simulink model "satellite3"  (R2025b)
settings: Solver=FixedStepAuto  StartTime=0.0  StopTime=100  FixedStep=dt  MinStep=0.0001  RelTol=1e-3
values from neighbouring files (symbols this model uses):
  A_mw = [ ... (first row only)    [init_params.m]
  A_w = [ ... (first row only)    [init_params.m]
  alpha1 = 0.1    [init_params.m]
  alpha2 = 0.1    [init_params.m]
  angle0 = eAR'    [init_params.m]
  area_d = 4    [init_params.m]
  area_m2 = 0.0127    [init_params.m]
  area_s = 2    [init_params.m]
  ARW_deg_per_sqrt_h = 0.01    [init_params.m]
  B_mw = [ ... (first row only)    [init_params.m]
  bat_bias_on = 0    [init_params.m]
  bat_bias_time = 0    [init_params.m]
  bat_bias_value = 0    [init_params.m]
  bat_cap_on = 0    [init_params.m]
  bat_cap_time = 0    [init_params.m]
  bat_cap_value = 1    [init_params.m]
  beta = 0.3    [init_params.m]
  beta1 = 0.01    [init_params.m]
  beta2 = 0.01    [init_params.m]
  bias0_deg_h = 0.01    [init_params.m]
  C_mw = [ ... (first row only)    [init_params.m]
  Cd = 2.2    [init_params.m]
  Cm = 0.01    [init_params.m]
  cmd_comm = 1    [init_params.m]
  comm_allow = 1    [init_params.m]
  cos_g_max = cos(gamma_max)    [init_params.m]
  Cr = 1.2    [init_params.m]
  cT_deg_on = 0    [init_params.m]
  cT_deg_time = 0    [init_params.m]
  cT_deg_value = 1    [init_params.m]
  cT_delay_on = 0    [init_params.m]
  cT_delay_time = 0    [init_params.m]
  cT_delay_value = 0    [init_params.m]
  cT_drop_on = 0    [init_params.m]
  cT_drop_time = 0    [init_params.m]
  cT_drop_value = 0    [init_params.m]
  cT_lock_on = 0    [init_params.m]
  cT_lock_time = 0    [init_params.m]
  d_c = 2e-5    (= 2e-05)    [init_params.m]
  d_f = 2e-5    (= 2e-05)    [init_params.m]
  D_max = 1    [init_params.m]
  D_thr = 0.4    [init_params.m]
  Delta_D = 0.001    [init_params.m]
  dP_th = 0.05    [init_params.m]
  dss_bias_on = 0    [init_params.m]
  dss_bias_time = 0    [init_params.m]
  dss_bias_value = [0;0;0]    [init_params.m]
  dss_delay_on = 0    [init_params.m]
  dss_delay_time = 0    [init_params.m]
  dss_delay_value = 0    [init_params.m]
  dss_drift_max = 0.1    [init_params.m]
  dss_drift_value = [0;0;0]    [init_params.m]
  dss_drop_on = 0    [init_params.m]
  dss_drop_time = 0    [init_params.m]
  dss_drop_value = [1;0;0]    [init_params.m]
  dss_lock_on = 0    [init_params.m]
  dss_lock_time = 0    [init_params.m]
  dt = 0.1    [init_params.m]
  earth_theta0 = 0    [init_params.m]
  epsilon = 0.01    [init_params.m]
  eT_deg_on = 0    [init_params.m]
  eT_deg_time = 0    [init_params.m]
  eT_deg_value = 1    [init_params.m]
  eT_delay_on = 0    [init_params.m]
  eT_delay_time = 0    [init_params.m]
  eT_delay_value = 0    [init_params.m]
  eT_drop_on = 0    [init_params.m]
  eT_drop_time = 0    [init_params.m]
  eT_drop_value = [0;0;0]    [init_params.m]
  eT_lock_on = 0    [init_params.m]
  eT_lock_time = 0    [init_params.m]
  eta = 0.7    [init_params.m]
  eta_buck = 0.9    [init_params.m]
  eta_et = 0.9    [init_params.m]
  eta_sspa = 0.35    [init_params.m]
  eta_twta = 0.35    [init_params.m]
  f = 2.2e9    (= 2200000000)    [init_params.m]
  f_n_hz = 400    [init_params.m]
  fov = 60*pi/180    (= 1.0471975512)    [init_params.m]
  g0 = 9.80665    [init_params.m]
  G0 = 1366.1    [init_params.m]
  G_sspa_dB = 20    [init_params.m]
  G_twta_dB = 20    [init_params.m]
  Gr_dB = 20    [init_params.m]
  Gt_dB = 3    [init_params.m]
  gyro_bias_on = 0    [init_params.m]
  gyro_bias_time = 0    [init_params.m]
  gyro_bias_value = [0;0;0]    [init_params.m]
  gyro_delay_on = 0    [init_params.m]
  gyro_delay_time = 0    [init_params.m]
  gyro_delay_value = 0    [init_params.m]
  gyro_drift_max = 0.1    [init_params.m]
  gyro_drift_value = [0;0;0]    [init_params.m]
  gyro_drop_on = 0    [init_params.m]
  gyro_drop_time = 0    [init_params.m]
  gyro_drop_value = [0;0;0]    [init_params.m]
  gyro_lock_on = 0    [init_params.m]
  gyro_lock_time = 0    [init_params.m]
  H = 50e3    (= 50000)    [init_params.m]
  h_max = Iw * rpm_max * sqrt(6)    [init_params.m]
  h_ref = 400e3    (= 400000)    [init_params.m]
  I_e = 11    [init_params.m]
  I_gate = 0.5    [init_params.m]
  I_triggle = 8    [init_params.m]
  i_w_max = 2    [init_params.m]
  i_w_min = -2    [init_params.m]
  initial_phase = 0    [init_params.m]
  Isp = 220    [init_params.m]
  Isp_et = 1500    [init_params.m]
  Iw = 0.02    [init_params.m]
  J2 = 1.08262668e-3    (= 0.00108262668)    [init_params.m]
  Jx = 10    [init_params.m]
  Jy = 12    [init_params.m]
  Jz = 8    [init_params.m]
  k_a = 4e-4    (= 0.0004)    [init_params.m]
  k_bias1_deg_h_per_C = 1    [init_params.m]
  k_bias2_deg_h_per_C = 0.0    (= 0)    [init_params.m]
  k_h = -0.05    [init_params.m]
  k_sf1_ppm = 1.0    (= 1)    [init_params.m]
  k_sf2_ppm = 0.0    (= 0)    [init_params.m]
  ... (+207 more)
libraries: matrix_library x25, simulink x14, nesl_utility x4, simulink_extras x3, fl_lib x3, ee_lib x1
(part 3 of 5)

== system satellite3/姿态确定与控制系统/三轴姿态动力学子系统/rlg_q/控模与扫模逻辑 ==
  光强 : Inport
  Add : Sum  Inputs=+-
  Add1 : Sum
  Gain : Gain  Gain=kP
  Gain1 : Gain  Gain=kI
  Integrator : Integrator
  Switch : Switch  Criteria=u2 > Threshold  SaturateOnIntegerOverflow=off  InputSameDT=off
  zero : Constant  Value=0  OutDataTypeStr=boolean
  光强阈值 : Constant  Value=I_triggle
  扫模信号发生器 : simulink/Sources/Repeating Sequence  rep_seq_t=[0 0.5 1]  rep_seq_y=[0 V_pzt_max V_pzt_min]
  期望光强 : Constant  Value=I_e
  状态切换 : simulink_extras/Flip Flops/S-R Flip-Flop  initial_condition=0
  触发信号 : RelationalOperator  OutDataTypeStr=boolean  RndMeth=Simplest  InputSameDT=off
  触发信号1 : RelationalOperator  Operator=<  OutDataTypeStr=boolean  RndMeth=Simplest  InputSameDT=off
  跌落阈值 : Constant  Value=I_gate
  扫模电压 : Outport
  wires:
  跌落阈值/1 -> 触发信号1/2
  光强/1 -> 触发信号/1, Add/2, 触发信号1/1
  触发信号1/1 -> 状态切换/2
  Integrator/1 -> Add1/1
  Gain1/1 -> Integrator/1
  Gain/1 -> Add1/2
  Add/1 -> Gain/1, Gain1/1
  Switch/1 -> 扫模电压/1
  触发信号/1 -> 状态切换/1
  扫模信号发生器/1 -> Switch/3
  状态切换/1 -> Switch/2
  Add1/1 -> Switch/1
  期望光强/1 -> Add/1
  光强阈值/1 -> 触发信号/2

== system satellite3/姿态确定与控制系统/三轴姿态动力学子系统/rlg_q/机械抖动 ==
  Add : Sum
  Add1 : Sum  Inputs=-+-
  Clock : Clock
  Product{,1..3,5} (5 alike) : Product
  Product6 : Product  Inputs=3
  Scope : Scope
      settings: DataLoggingVariableName=ScopeData4
  Scope1 : Scope
      settings: DataLoggingVariableName=ScopeData5
  Sin : Trigonometry
  Square : Math  Operator=square
  deg2rad : Gain  Gain=pi/180
  dither_d : ToWorkspace  VariableName=dither_d  SampleTime=-1
  dither_w : ToWorkspace  VariableName=dither_w  SampleTime=-1
  r2rad : Gain  Gain=2*pi
  倍数 : Constant  Value=2.0
  初相位 : Constant  Value=initial_phase
  抖动固有频率-Hz : Constant  Value=f_n_hz
  抖动角度迭代 : Integrator
  抖动角速度迭代 : Integrator
  抖动角速度（峰值）-deg/s : Constant  Value=v_peak_deg_s
  阻尼比 : Constant  Value=zeta
  抖动角速度 : Outport
  wires:
  抖动角速度迭代/1 -> 抖动角度迭代/1, 抖动角速度/1, Product6/3, dither_w/1, Scope/1
  Product5/1 -> Add1/1
  抖动角度迭代/1 -> Product5/1, Scope1/1, dither_d/1
  Square/1 -> Product5/2
  Product6/1 -> Add1/3
  Add1/1 -> 抖动角速度迭代/1
  Product/1 -> Product3/2, Product6/2
  抖动角速度（峰值）-deg/s/1 -> deg2rad/1
  deg2rad/1 -> Product3/1  "抖动角度幅值-rad"
  Product2/1 -> Add1/2  "驱动力矩-N·m"
  Sin/1 -> Product2/2
  Product3/1 -> Product2/1  "驱动力矩幅值-N·m"
  Add/1 -> Sin/1
  初相位/1 -> Add/2
  Product1/1 -> Add/1
  Clock/1 -> Product1/1
  倍数/1 -> Product/1
  阻尼比/1 -> Product/2
  抖动固有频率-Hz/1 -> r2rad/1
  r2rad/1 -> Product1/2, Product6/1, Square/1  "抖动固有角频率-rad/s"

== system satellite3/姿态确定与控制系统/三轴姿态动力学子系统/rlg_q/热模型 ==
  环境温度-°C : Inport
  几何标度因数 : Inport  Port=2
  Add : Sum
  Add1 : Sum  Inputs=+++
  Add2 : Sum
  Product : Product
  Sum : Sum  Inputs=|-+
  deg2rad(s) : Gain  Gain=pi/(180*3600)
  平方 : Math  Operator=square
  标定/初始温度 : Constant  Value=25
  标度因数倍数（参考温度） : Constant
  比较 : Sum  Inputs=-+|
  温度标度因数系数（1阶） : Gain  Gain=k_sf1_ppm
  温度标度因数系数（2阶） : Gain  Gain=k_sf2_ppm
  温度迭代 : Integrator  InitialConditionSource=external  InitialCondition=25.0
  温度零偏系数（1阶） : Gain  Gain=k_bias1_deg_h_per_C
  温度零偏系数（2阶） : Gain  Gain=k_bias2_deg_h_per_C
  热时间常数 : Gain  Gain=1/tau_th_s
  百万分之一每摄氏度 : Gain  Gain=1e-6
  零偏（参考温度） : Constant  Value=bias0_deg_h
  陀螺温度-°C : Outport
  温度标度因数 : Outport  Port=2
  温度零偏 : Outport  Port=3
  wires:
  Add2/1 -> Product/2
  标度因数倍数（参考温度）/1 -> Add2/1
  百万分之一每摄氏度/1 -> Add2/2
  零偏（参考温度）/1 -> Add1/1
  温度零偏系数（1阶）/1 -> Add1/2
  温度零偏系数（2阶）/1 -> Add1/3
  Sum/1 -> 温度零偏系数（1阶）/1, 温度标度因数系数（1阶）/1, 平方/1
  Add1/1 -> deg2rad(s)/1
  几何标度因数/1 -> Product/1
  deg2rad(s)/1 -> 温度零偏/1
  平方/1 -> 温度零偏系数（2阶）/1, 温度标度因数系数（2阶）/1
  Product/1 -> 温度标度因数/1
  Add/1 -> 百万分之一每摄氏度/1
  标定/初始温度/1 -> 温度迭代/2, Sum/1
  温度标度因数系数（2阶）/1 -> Add/2
  温度标度因数系数（1阶）/1 -> Add/1
  比较/1 -> 热时间常数/1
  环境温度-°C/1 -> 比较/2
  温度迭代/1 -> 比较/1, Sum/2, 陀螺温度-°C/1
  热时间常数/1 -> 温度迭代/1

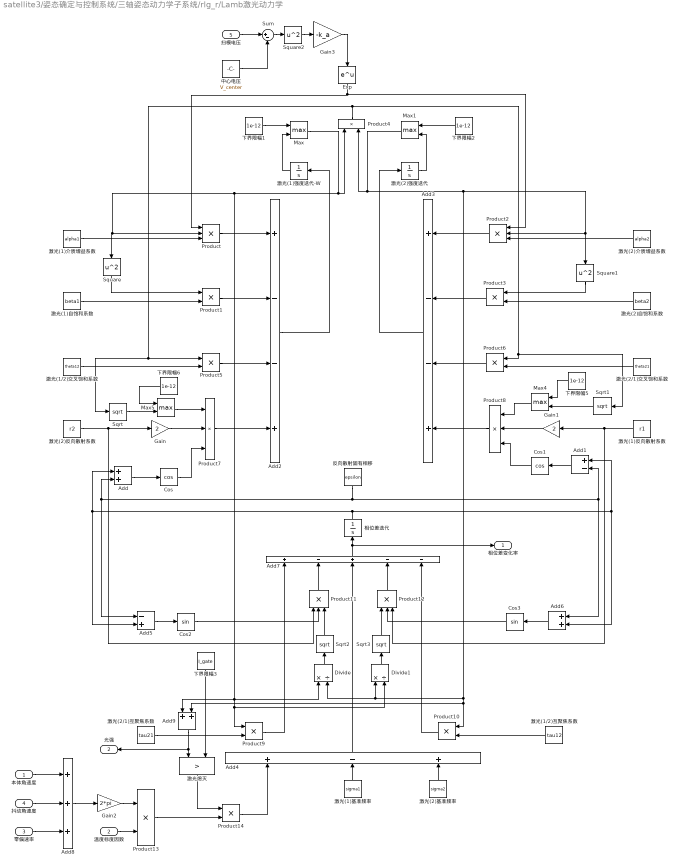
== system satellite3/姿态确定与控制系统/三轴姿态动力学子系统/rlg_r/Lamb激光动力学 ==
  本体角速度 : Inport
  温度标度因数 : Inport  Port=2
  零偏速率 : Inport  Port=3
  抖动角速度 : Inport  Port=4
  扫模电压 : Inport  Port=5
  Add : Sum
  Add1 : Sum  Inputs=+-
  Add2 : Sum  Inputs=+--+
  Add3 : Sum  Inputs=+--+
  Add4 : Sum  Inputs=+-+
  Add5 : Sum  Inputs=-+
  Add6 : Sum
  Add7 : Sum  Inputs=+-+--
  Add8 : Sum  Inputs=+++
  Add9 : Sum
  Cos : Trigonometry  Operator=cos
  Cos1 : Trigonometry  Operator=cos
  Cos2 : Trigonometry
  Cos3 : Trigonometry
  Divide : Product  Inputs=*/
  Divide1 : Product  Inputs=*/
  Exp : Math
  Gain : Gain  Gain=2
  Gain1 : Gain  Gain=2
  Gain2 : Gain  Gain=2*pi
  Gain3 : Gain  Gain=-k_a
  Max{,1,4..5} (4 alike) : MinMax  Function=max  Inputs=2
  Product{,2,7..8,11..12} (6 alike) : Product  Inputs=3
  Product{1,3..6,9..10,13..14} (9 alike) : Product
  Sqrt{,1..3} (4 alike) : Sqrt
  Square : Math  Operator=square
  Square1 : Math  Operator=square
  Square2 : Math  Operator=square
  Sum : Sum  Inputs=|+-
  下界限幅{1..2,5..6} (4 alike) : Constant  Value=1e-12
  下界限幅3 : Constant  Value=I_gate
  中心电压 : Constant  Value=V_center
  反向散射固有相移 : Constant  Value=epsilon
  激光(1)介质增益系数 : Constant  Value=alpha1
  激光(1)反向散射系数 : Constant  Value=r1
  激光(1)基准频率 : Constant  Value=sigma1
  激光(1)强度迭代-W : Integrator  InitialCondition=1
  激光(1)自饱和系数 : Constant  Value=beta1
  激光(1/2)互聚焦系数 : Constant  Value=tau12
  激光(1/2)交叉饱和系数 : Constant  Value=theta12
  激光(2)介质增益系数 : Constant  Value=alpha2
  激光(2)反向散射系数 : Constant  Value=r2
  激光(2)基准频率 : Constant  Value=sigma2
  激光(2)强度迭代 : Integrator  InitialCondition=1
  激光(2)自饱和系数 : Constant  Value=beta2
  激光(2/1)互聚焦系数 : Constant  Value=tau21
  激光(2/1)交叉饱和系数 : Constant  Value=theta21
  激光熄灭 : RelationalOperator  Operator=>  OutDataTypeStr=boolean  InputSameDT=off
  相位差迭代 : Integrator
  相位差变化率 : Outport
  光强 : Outport  Port=2
  wires:
  激光(1)介质增益系数/1 -> Product/3
  激光(1)自饱和系数/1 -> Product1/2
  Square/1 -> Product1/1
  激光(2)介质增益系数/1 -> Product2/3
  激光(2)自饱和系数/1 -> Product3/2
  Square1/1 -> Product3/1
  激光(1/2)交叉饱和系数/1 -> Product5/2
  激光(2/1)交叉饱和系数/1 -> Product6/2
  下界限幅1/1 -> Max/1
  Product4/1 -> Product6/1, Sqrt1/1, Product5/1, Sqrt/1
  激光(2)反向散射系数/1 -> Gain/1, Product11/1
  Gain/1 -> Product7/2
  Max5/1 -> Product7/1
  Cos/1 -> Product7/3
  Add/1 -> Cos/1
  反向散射固有相移/1 -> Add1/2, Add6/1, Add5/1, Add/2
  Cos1/1 -> Product8/3
  Max4/1 -> Product8/1
  Add1/1 -> Cos1/1
  Gain1/1 -> Product8/2
  激光(1)反向散射系数/1 -> Product12/3, Gain1/1
  下界限幅2/1 -> Max1/1
  Product/1 -> Add2/1
  Product1/1 -> Add2/2
  Product5/1 -> Add2/3
  Add2/1 -> 激光(1)强度迭代-W/1
  Product2/1 -> Add3/1
  Product3/1 -> Add3/2
  Product6/1 -> Add3/3
  Product8/1 -> Add3/4
  Add3/1 -> 激光(2)强度迭代/1
  激光(2/1)互聚焦系数/1 -> Product9/2
  激光(1/2)互聚焦系数/1 -> Product10/2
  Product7/1 -> Add2/4
  Add5/1 -> Cos2/1
  Max/1 -> Add9/1, Product9/1, Divide1/2, Divide/1, Product/2, Square/1, Product4/1
  Divide/1 -> Sqrt2/1
  Cos2/1 -> Product11/2
  相位差迭代/1 -> Add1/1, Add6/2, Add5/2, Add/1
  Add6/1 -> Cos3/1
  Divide1/1 -> Sqrt3/1
  Cos3/1 -> Product12/2
  激光(1)基准频率/1 -> Add4/2
  激光(2)基准频率/1 -> Add4/3
  Product14/1 -> Add4/1
  Product9/1 -> Add7/1
  Product10/1 -> Add7/5
  Product11/1 -> Add7/2
  Product12/1 -> Add7/4
  Add4/1 -> Add7/3
  Add7/1 -> 相位差变化率/1, 相位差迭代/1
  激光(1)强度迭代-W/1 -> Max/2
  激光(2)强度迭代/1 -> Max1/2
  下界限幅5/1 -> Max4/1
  Sqrt1/1 -> Max4/2
  下界限幅6/1 -> Max5/1
  Sqrt/1 -> Max5/2
  Sqrt2/1 -> Product11/3
  Sqrt3/1 -> Product12/1
  零偏速率/1 -> Add8/3
  温度标度因数/1 -> Product13/2
  本体角速度/1 -> Add8/1
  抖动角速度/1 -> Add8/2
  Add8/1 -> Gain2/1
  Gain2/1 -> Product13/1
  Max1/1 -> Product4/2, Square1/1, Product2/2, Divide/2, Divide1/1, Add9/2, Product10/1
  Add9/1 -> 光强/1, 激光熄灭/1
  Product13/1 -> Product14/2
  激光熄灭/1 -> Product14/1
  下界限幅3/1 -> 激光熄灭/2
  扫模电压/1 -> Sum/1
  中心电压/1 -> Sum/2
  Sum/1 -> Square2/1
  Gain3/1 -> Exp/1
  Exp/1 -> Product2/1, Product/1
  Square2/1 -> Gain3/1

== system satellite3/姿态确定与控制系统/三轴姿态动力学子系统/rlg_r/几何参数 ==
  Mux : Mux  Inputs=3
  激光波长-m : Constant  Value=wavelength_m
  环形腔周长-m : Constant  Value=perimeter_m
  环形腔面积-m2 : Constant  Value=area_m2
  计算集合标度因数-S0 : Fcn  Expr=4*u(1)/(u(2)*u(3))
  标度因数 : Outport
  wires:
  计算集合标度因数-S0/1 -> 标度因数/1
  Mux/1 -> 计算集合标度因数-S0/1
  环形腔面积-m2/1 -> Mux/1
  激光波长-m/1 -> Mux/2
  环形腔周长-m/1 -> Mux/3

== system satellite3/姿态确定与控制系统/三轴姿态动力学子系统/rlg_r/噪声模型 ==
  标度因数 : Inport
  相位差变化率 : Inport  Port=2
  Add : Sum
  Band-Limited White Noise : simulink/Sources/Band-Limited White Noise  Cov=[(ARW_deg_per_sqrt_h/60)^2 + white_rate_std_deg_s^2]  Ts=1  seed=[23341]
  Divide : Product  Inputs=/*
  Gain : Gain  Gain=pi/180
  r2Hz : Gain  Gain=1/(2*pi)
  测量角速度 : Outport
  wires:
  Add/1 -> 测量角速度/1
  r2Hz/1 -> Divide/2
  Gain/1 -> Add/1
  Band-Limited White Noise/1 -> Gain/1
  Divide/1 -> Add/2
  相位差变化率/1 -> r2Hz/1
  标度因数/1 -> Divide/1

== system satellite3/姿态确定与控制系统/三轴姿态动力学子系统/rlg_r/控模与扫模逻辑 ==
  光强 : Inport
  Add : Sum  Inputs=+-
  Add1 : Sum
  Gain : Gain  Gain=kP
  Gain1 : Gain  Gain=kI
  Integrator : Integrator
  Switch : Switch  Criteria=u2 > Threshold  SaturateOnIntegerOverflow=off  InputSameDT=off
  zero : Constant  Value=0  OutDataTypeStr=boolean
  光强阈值 : Constant  Value=I_triggle
  扫模信号发生器 : simulink/Sources/Repeating Sequence  rep_seq_t=[0 0.5 1]  rep_seq_y=[0 V_pzt_max V_pzt_min]
  期望光强 : Constant  Value=I_e
  状态切换 : simulink_extras/Flip Flops/S-R Flip-Flop  initial_condition=0
  触发信号 : RelationalOperator  OutDataTypeStr=boolean  RndMeth=Simplest  InputSameDT=off
  触发信号1 : RelationalOperator  Operator=<  OutDataTypeStr=boolean  RndMeth=Simplest  InputSameDT=off
  跌落阈值 : Constant  Value=I_gate
  扫模电压 : Outport
  wires:
  光强阈值/1 -> 触发信号/2
  期望光强/1 -> Add/1
  Add1/1 -> Switch/1
  状态切换/1 -> Switch/2
  扫模信号发生器/1 -> Switch/3
  触发信号/1 -> 状态切换/1
  Switch/1 -> 扫模电压/1
  Add/1 -> Gain1/1, Gain/1
  Gain/1 -> Add1/2
  Gain1/1 -> Integrator/1
  Integrator/1 -> Add1/1
  触发信号1/1 -> 状态切换/2
  光强/1 -> 触发信号1/1, Add/2, 触发信号/1
  跌落阈值/1 -> 触发信号1/2

== system satellite3/姿态确定与控制系统/三轴姿态动力学子系统/rlg_r/机械抖动 ==
  Add : Sum
  Add1 : Sum  Inputs=-+-
  Clock : Clock
  Product{,1..3,5} (5 alike) : Product
  Product6 : Product  Inputs=3
  Scope : Scope
      settings: DataLoggingVariableName=ScopeData4
  Scope1 : Scope
      settings: DataLoggingVariableName=ScopeData5
  Sin : Trigonometry
  Square : Math  Operator=square
  deg2rad : Gain  Gain=pi/180
  dither_d : ToWorkspace  VariableName=dither_d  SampleTime=-1
  dither_w : ToWorkspace  VariableName=dither_w  SampleTime=-1
  r2rad : Gain  Gain=2*pi
  倍数 : Constant  Value=2.0
  初相位 : Constant  Value=initial_phase
  抖动固有频率-Hz : Constant  Value=f_n_hz
  抖动角度迭代 : Integrator
  抖动角速度迭代 : Integrator
  抖动角速度（峰值）-deg/s : Constant  Value=v_peak_deg_s
  阻尼比 : Constant  Value=zeta
  抖动角速度 : Outport
  wires:
  r2rad/1 -> Square/1, Product6/1, Product1/2  "抖动固有角频率-rad/s"
  抖动固有频率-Hz/1 -> r2rad/1
  阻尼比/1 -> Product/2
  倍数/1 -> Product/1
  Clock/1 -> Product1/1
  Product1/1 -> Add/1
  初相位/1 -> Add/2
  Add/1 -> Sin/1
  Product3/1 -> Product2/1  "驱动力矩幅值-N·m"
  Sin/1 -> Product2/2
  Product2/1 -> Add1/2  "驱动力矩-N·m"
  deg2rad/1 -> Product3/1  "抖动角度幅值-rad"
  抖动角速度（峰值）-deg/s/1 -> deg2rad/1
  Product/1 -> Product6/2, Product3/2
  Add1/1 -> 抖动角速度迭代/1
  Product6/1 -> Add1/3
  Square/1 -> Product5/2
  抖动角度迭代/1 -> dither_d/1, Scope1/1, Product5/1
  Product5/1 -> Add1/1
  抖动角速度迭代/1 -> Scope/1, dither_w/1, Product6/3, 抖动角速度/1, 抖动角度迭代/1

== system satellite3/姿态确定与控制系统/三轴姿态动力学子系统/rlg_r/热模型 ==
  环境温度-°C : Inport
  几何标度因数 : Inport  Port=2
  Add : Sum
  Add1 : Sum  Inputs=+++
  Add2 : Sum
  Product : Product
  Sum : Sum  Inputs=|-+
  deg2rad(s) : Gain  Gain=pi/(180*3600)
  平方 : Math  Operator=square
  标定/初始温度 : Constant  Value=25
  标度因数倍数（参考温度） : Constant
  比较 : Sum  Inputs=-+|
  温度标度因数系数（1阶） : Gain  Gain=k_sf1_ppm
  温度标度因数系数（2阶） : Gain  Gain=k_sf2_ppm
  温度迭代 : Integrator  InitialConditionSource=external  InitialCondition=25.0
  温度零偏系数（1阶） : Gain  Gain=k_bias1_deg_h_per_C
  温度零偏系数（2阶） : Gain  Gain=k_bias2_deg_h_per_C
  热时间常数 : Gain  Gain=1/tau_th_s
  百万分之一每摄氏度 : Gain  Gain=1e-6
  零偏（参考温度） : Constant  Value=bias0_deg_h
  陀螺温度-°C : Outport
  温度标度因数 : Outport  Port=2
  温度零偏 : Outport  Port=3
  wires:
  热时间常数/1 -> 温度迭代/1
  温度迭代/1 -> 陀螺温度-°C/1, Sum/2, 比较/1
  环境温度-°C/1 -> 比较/2
  比较/1 -> 热时间常数/1
  温度标度因数系数（1阶）/1 -> Add/1
  温度标度因数系数（2阶）/1 -> Add/2
  标定/初始温度/1 -> Sum/1, 温度迭代/2
  Add/1 -> 百万分之一每摄氏度/1
  Product/1 -> 温度标度因数/1
  平方/1 -> 温度标度因数系数（2阶）/1, 温度零偏系数（2阶）/1
  deg2rad(s)/1 -> 温度零偏/1
  几何标度因数/1 -> Product/1
  Add1/1 -> deg2rad(s)/1
  Sum/1 -> 平方/1, 温度标度因数系数（1阶）/1, 温度零偏系数（1阶）/1
  温度零偏系数（2阶）/1 -> Add1/3
  温度零偏系数（1阶）/1 -> Add1/2
  零偏（参考温度）/1 -> Add1/1
  百万分之一每摄氏度/1 -> Add2/2
  标度因数倍数（参考温度）/1 -> Add2/1
  Add2/1 -> Product/2

== system satellite3/姿态确定与控制系统/三轴姿态动力学子系统/四元数传播-闭式积分/向量模长-r ==
  u1 : Inport
  Add : Sum  Inputs=+++
  Demux : Demux  Outputs=3
  Sqrt : Sqrt
  Square : Math  Operator=square
  Square1 : Math  Operator=square
  Square2 : Math  Operator=square
  |u| : Outport
  wires:
  Demux/1 -> Square/1
  Demux/2 -> Square1/1
  Demux/3 -> Square2/1
  Square/1 -> Add/1
  Square1/1 -> Add/2
  Square2/1 -> Add/3
  Add/1 -> Sqrt/1
  Sqrt/1 -> |u|/1
  u1/1 -> Demux/1

== system satellite3/姿态确定与控制系统/三轴姿态动力学子系统/四元数传播-闭式积分/四元数乘法 ==
  Q1 : Inport
  Q2 : Inport  Port=2
  Add : Sum  Inputs=3
  Cross Product : matrix_library/Cross Product
  Demux : Demux
  Demux1 : Demux
  Dot Product : DotProduct  OutDataTypeStr=Inherit: Inherit via internal rule
  Mux : Mux  Inputs=2
  Mux1 : Mux  Inputs=3
  Mux2 : Mux  Inputs=3
  Product : Product
  Product1 : Product
  Product2 : Product
  Sum : Sum  Inputs=|+-
  Q* : Outport
  wires:
  Q1/1 -> Demux/1
  Q2/1 -> Demux1/1
  Mux/1 -> Q*/1
  Product/1 -> Sum/1
  Demux/1 -> Product1/1, Product/1
  Mux1/1 -> Dot Product/1, Cross Product/1, Product2/2
  Demux1/1 -> Product2/1, Product/2
  Mux2/1 -> Cross Product/2, Dot Product/2, Product1/2
  Sum/1 -> Mux/1
  Dot Product/1 -> Sum/2
  Product2/1 -> Add/2
  Product1/1 -> Add/1
  Cross Product/1 -> Add/3
  Add/1 -> Mux/2
  Demux/2 -> Mux1/1
  Demux/3 -> Mux1/2
  Demux/4 -> Mux1/3
  Demux1/2 -> Mux2/1
  Demux1/3 -> Mux2/2
  Demux1/4 -> Mux2/3

== system satellite3/姿态确定与控制系统/三轴姿态动力学子系统/四元数传播-闭式积分/四元数乘法1 ==
  Q1 : Inport
  Q2 : Inport  Port=2
  Add : Sum  Inputs=3
  Cross Product : matrix_library/Cross Product
  Demux : Demux
  Demux1 : Demux
  Dot Product : DotProduct  OutDataTypeStr=Inherit: Inherit via internal rule
  Mux : Mux  Inputs=2
  Mux1 : Mux  Inputs=3
  Mux2 : Mux  Inputs=3
  Product : Product
  Product1 : Product
  Product2 : Product
  Sum : Sum  Inputs=|+-
  Q* : Outport
  wires:
  Q1/1 -> Demux/1
  Q2/1 -> Demux1/1
  Mux/1 -> Q*/1
  Product/1 -> Sum/1
  Demux/1 -> Product1/1, Product/1
  Mux1/1 -> Dot Product/1, Cross Product/1, Product2/2
  Demux1/1 -> Product2/1, Product/2
  Mux2/1 -> Cross Product/2, Dot Product/2, Product1/2
  Sum/1 -> Mux/1
  Dot Product/1 -> Sum/2
  Product2/1 -> Add/2
  Product1/1 -> Add/1
  Cross Product/1 -> Add/3
  Add/1 -> Mux/2
  Demux/2 -> Mux1/1
  Demux/3 -> Mux1/2
  Demux/4 -> Mux1/3
  Demux1/2 -> Mux2/1
  Demux1/3 -> Mux2/2
  Demux1/4 -> Mux2/3

== system satellite3/姿态确定与控制系统/三轴姿态动力学子系统/姿态解算/四元数传播-欧拉法 ==
  note: $\dot{q}=\frac{1}{2} \left[\begin{array}{ccc} -q_1&-q_2&-q_3 \\ q_0&-q_3&q_2\\ q_3&q_0&-q_1\\ -q_2&q_1&q_0 \end{array}\right]\omega$
  机体系角速度分量 : Inport
  Demux : Demux
  Int_q0 : Integrator  InitialCondition=Q0(1)
  Int_q1 : Integrator  InitialCondition=Q0(2)
  Int_q2 : Integrator  InitialCondition=Q0(3)
  Int_q3 : Integrator  InitialCondition=Q0(4)
  Mux : Mux
  Product : Product  Multiplication=Matrix(*)
  Product{1..4} (4 alike) : Product  Inputs=*/
  Transpose : Math  Operator=transpose
  Vector Concatenate : Concatenate  NumInputs=4  Mode=Multidimensional array  ConcatenateDimension=2
  neg1 : Gain  Gain=-1
  neg2 : Gain  Gain=-1
  neg3 : Gain  Gain=-1
  q0_dot : Mux  Inputs=3
  q1_dot : Mux  Inputs=3
  q1_dot1 : Mux  Inputs=3
  q1_dot2 : Mux  Inputs=3
  向量模长-q : Subsystem
  四元数 : Outport
  wires:
  Product/1 -> Demux/1
  neg1/1 -> q0_dot/1, q1_dot1/3
  q1_dot/1 -> Vector Concatenate/2
  neg3/1 -> q1_dot/2, q0_dot/3
  Product4/1 -> neg3/1, Mux/4, q1_dot1/1  "q3"
  Product1/1 -> q1_dot/1, q1_dot1/2, Mux/1, q1_dot2/3  "q0"
  q1_dot1/1 -> Vector Concatenate/3
  Demux/2 -> Int_q1/1
  Product2/1 -> neg1/1, Mux/2, q1_dot2/2  "q1"
  Demux/3 -> Int_q2/1
  neg2/1 -> q1_dot2/1, q0_dot/2
  q1_dot2/1 -> Vector Concatenate/4
  Product3/1 -> neg2/1, Mux/3, q1_dot/3  "q2"
  q0_dot/1 -> Vector Concatenate/1
  Vector Concatenate/1 -> Transpose/1
  Demux/1 -> Int_q0/1
  Demux/4 -> Int_q3/1
  机体系角速度分量/1 -> Product/2
  Transpose/1 -> Product/1
  Int_q0/1 -> Product1/1, 向量模长-q/1(u0)
  Int_q1/1 -> Product2/1, 向量模长-q/2(u1)
  Int_q2/1 -> Product3/1, 向量模长-q/3(u2)
  Int_q3/1 -> Product4/1, 向量模长-q/4(u3)
  向量模长-q/1(|u|) -> Product2/2, Product3/2, Product4/2, Product1/2
  Mux/1 -> 四元数/1

== system satellite3/姿态确定与控制系统/三轴姿态动力学子系统/姿态解算/星敏 ==
  note: 调试先用pulse，再考虑换为0~1均匀分布
  q_true : Inport
  valid_cmd : Inport  Port=2
  Pulse Generator : DiscretePulseGenerator  PulseType=Time based  Period=10  PulseWidth=90
  Relational Operator : RelationalOperator  Operator=<=  OutDataTypeStr=boolean  RndMeth=Simplest  InputSameDT=off
  Uniform Random Number : UniformRandomNumber  Minimum=0  SampleTime=0.1
  delay : TransportDelay  DelayTime=T_delay_st  InitialOutput=[Q0(1);Q0(2);Q0(3);Q0(4)]
  sample : ZeroOrderHold  SampleTime=Ts_st
  四元数乘法 : Subsystem
  四元数归一化 : Subsystem
  掉帧概率 : Constant  Value=p_drop
  误差四元数 : Subsystem
  q_star : Outport
  st_valid : Outport  Port=2
  wires:
  q_true/1 -> sample/1
  sample/1 -> delay/1
  四元数归一化/1(Out1) -> q_star/1
  delay/1 -> 四元数乘法/1(Q1)
  误差四元数/1(delta_q) -> 四元数乘法/2(Q2)
  四元数乘法/1(Q*) -> 四元数归一化/1(Q*)
  掉帧概率/1 -> Relational Operator/2
  Uniform Random Number/1 -> Relational Operator/1
  Pulse Generator/1 -> st_valid/1

== system satellite3/姿态确定与控制系统/三轴姿态动力学子系统/姿态解算/欧拉数传播 ==
  机体系角速度分量 : Inport
  Demux : Demux  Outputs=3
  Gain : Gain  Gain=-1
  Int_phi : Integrator  InitialCondition=angle0(1)
  Int_psi : Integrator  InitialCondition=angle0(3)
  Int_theta : Integrator  InitialCondition=angle0(2)
  Mux{,1..3} (4 alike) : Mux  Inputs=3
  Product : Product  Inputs=**/
  Product1 : Product  Inputs=**/
  Product2 : Product  Inputs=*/
  Product3 : Product  Inputs=/*
  Product4 : Product  Multiplication=Matrix(*)
  Sin1 : Trigonometry
  Sin2 : Trigonometry
  Sin3 : Trigonometry  Operator=cos
  Sin4 : Trigonometry  Operator=cos
  Transpose : Math  Operator=transpose
  Vector Concatenate : Concatenate  NumInputs=3  Mode=Multidimensional array  ConcatenateDimension=2
  三轴欧拉角 : Outport
  wires:
  Mux2/1 -> Vector Concatenate/3
  Gain/1 -> Mux1/3
  Demux/1 -> Int_phi/1
  [one] -> Mux/1
  Demux/3 -> Int_psi/1
  Demux/2 -> Int_theta/1
  Product1/1 -> Mux/3
  Int_theta/1 -> Mux3/2, Sin3/1, Sin1/1  "theta"
  Mux/1 -> Vector Concatenate/1
  Mux1/1 -> Vector Concatenate/2
  Product3/1 -> Mux2/3
  Vector Concatenate/1 -> Transpose/1
  Product2/1 -> Mux2/2
  [zero] -> Mux2/1, Mux1/1
  机体系角速度分量/1 -> Product4/2
  Product/1 -> Mux/2
  Product4/1 -> Demux/1
  Int_phi/1 -> Sin4/1, Sin2/1, Mux3/1  "phi"
  Mux3/1 -> 三轴欧拉角/1
  Int_psi/1 -> Mux3/3
  Sin2/1 -> Gain/1, Product2/1, Product/1
  Sin1/1 -> Product1/2, Product/2
  Sin3/1 -> Product3/1, Product2/2, Product1/3, Product/3
  Sin4/1 -> Product3/2, Product1/1, Mux1/2
  Transpose/1 -> Product4/1

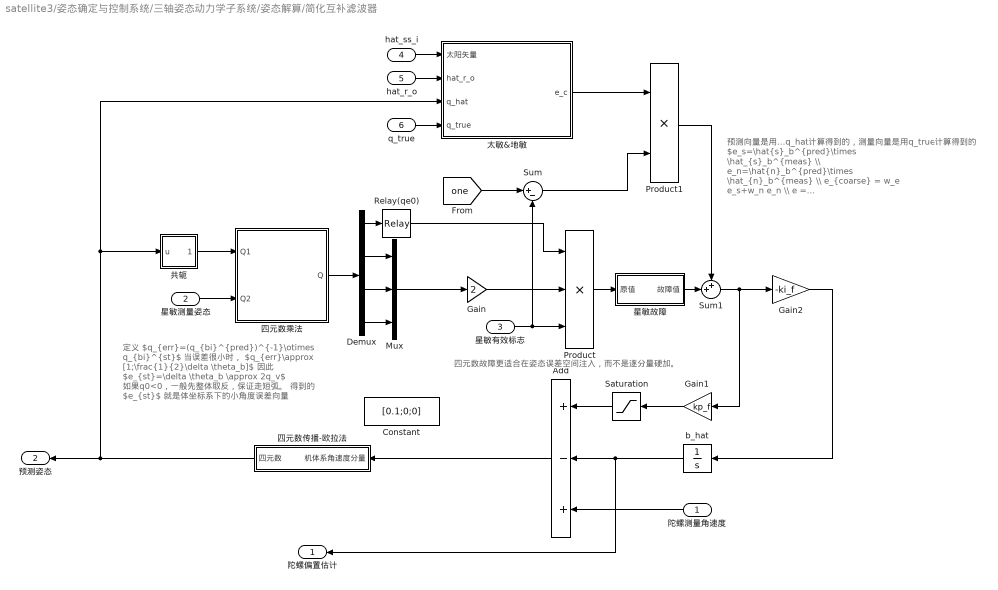
== system satellite3/姿态确定与控制系统/三轴姿态动力学子系统/姿态解算/简化互补滤波器 ==
  note: 定义 $q_{err}=(q_{bi}^{pred})^{-1}\otimes q_{bi}^{st}$
      | 当误差很小时， $q_{err}\approx [1;\frac{1}{2}\delta \theta_b]$
      | 因此 $e_{st}=\delta \theta_b \approx 2q_v$
      | 如果q0<0，一般先整体取反，保证走短弧。
      | 得到的 $e_{st}$ 就是体坐标系下的小角度误差向量
  note: 四元数故障更适合在姿态误差空间注入，而不是逐分量硬加。
  note: 预测向量是用q_hat计算得到的，测量向量是用q_true计算得到的
      | $e_s=\hat{s}_b^{pred}\times \hat_{s}_b^{meas} \\ e_n=\hat{n}_b^{pred}\times \hat_{n}_b^{meas} \\ e_{coarse} = w_e e_s+w_n e_n \\ e = st\_valid*e_{st}+(1-st\_valid)*e_{coarse}$
      | 但由于地敏简化，解算值与测量值相同
  陀螺测量角速度 : Inport
  星敏测量姿态 : Inport  Port=2
  星敏有效标志 : Inport  Port=3
  hat_ss_i : Inport  Port=4
  hat_r_o : Inport  Port=5
  q_true : Inport  Port=6
  Add : Sum  Inputs=+-+
  Constant : Constant  Value=[0.1;0;0]
  Demux : Demux
  Gain : Gain  Gain=2
  Gain1 : Gain  Gain=kp_f
  Gain2 : Gain  Gain=-ki_f
  Mux : Mux  Inputs=3
  Product : Product  Inputs=3
  Product1 : Product
  Relay(qe0) : Relay  OffOutputValue=-1
  Saturation : Saturate  UpperLimit=Tcorr_limit  LowerLimit=-Tcorr_limit
  Sum : Sum  Inputs=|+-
  Sum1 : Sum  Inputs=++|
  b_hat : Integrator  InitialCondition=[0;0;0]
  共轭 : Subsystem
  四元数乘法 : Subsystem
  四元数传播-欧拉法 : Subsystem
  太敏&地敏 : Subsystem
  星敏故障 : Subsystem
  陀螺偏置估计 : Outport
  预测姿态 : Outport  Port=2
  wires:
  四元数传播-欧拉法/1(四元数) -> 预测姿态/1, 太敏&地敏/3(q_hat), 共轭/1(u)
  共轭/1(u^-1) -> 四元数乘法/1(Q1)
  星敏测量姿态/1 -> 四元数乘法/2(Q2)
  Demux/2 -> Mux/1
  Relay(qe0)/1 -> Product/1
  Demux/1 -> Relay(qe0)/1
  Mux/1 -> Gain/1
  Demux/4 -> Mux/3
  Demux/3 -> Mux/2
  四元数乘法/1(Q) -> Demux/1
  Gain/1 -> Product/2
  星敏有效标志/1 -> Product/3, Sum/2
  b_hat/1 -> 陀螺偏置估计/1, Add/2
  陀螺测量角速度/1 -> Add/3
  Gain1/1 -> Saturation/1
  Saturation/1 -> Add/1
  Sum1/1 -> Gain2/1, Gain1/1
  Gain2/1 -> b_hat/1
  Add/1 -> 四元数传播-欧拉法/1(机体系角速度分量)
  hat_ss_i/1 -> 太敏&地敏/1(太阳矢量)
  hat_r_o/1 -> 太敏&地敏/2(hat_r_o)
  q_true/1 -> 太敏&地敏/4(q_true)
  太敏&地敏/1(e_c) -> Product1/1
  [one] -> Sum/1
  Sum/1 -> Product1/2
  Product/1 -> 星敏故障/1(原值)
  Product1/1 -> Sum1/1
  星敏故障/1(故障值) -> Sum1/2

== system satellite3/姿态确定与控制系统/三轴姿态动力学子系统/陀螺仪故障/偏差故障 ==
  使能*幅度 : Gain  Gain=gyro_bias_on*gyro_bias_value
  注入时间 : Step  Time=gyro_bias_time  SampleTime=0
  故障值注入 : Outport
  wires:
  注入时间/1 -> 使能*幅度/1
  使能*幅度/1 -> 故障值注入/1

== system satellite3/姿态确定与控制系统/三轴姿态动力学子系统/陀螺仪故障/延迟故障 ==
  原值 : Inport
  Delay : Delay  DelayLength=gyro_delay_value
  Switch : Switch  Criteria=u2 > Threshold  Threshold=0.5  SaturateOnIntegerOverflow=off  InputSameDT=off
  使能 : Gain  Gain=gyro_delay_on
  抵消 : Sum  Inputs=|+-
  注入时间 : Step  Time=gyro_delay_time  SampleTime=0
  故障值注入 : Outport
  wires:
  使能/1 -> Switch/2
  注入时间/1 -> 使能/1
  原值/1 -> Delay/1, Switch/3, 抵消/2
  抵消/1 -> 故障值注入/1
  Switch/1 -> 抵消/1
  Delay/1 -> Switch/1

== system satellite3/姿态确定与控制系统/三轴姿态动力学子系统/陀螺仪故障/掉线故障 ==
  原值 : Inport
  Switch : Switch  Criteria=u2 > Threshold  Threshold=0.5  SaturateOnIntegerOverflow=off  InputSameDT=off
  Zero : Constant  Value=gyro_drop_value  OutDataTypeStr=Inherit: Inherit via back propagation
  使能 : Gain  Gain=gyro_drop_on
  抵消 : Sum  Inputs=|+-
  注入时间 : Step  Time=gyro_drop_time  SampleTime=0
  故障值注入 : Outport
  wires:
  Zero/1 -> Switch/1
  Switch/1 -> 抵消/1
  抵消/1 -> 故障值注入/1
  原值/1 -> 抵消/2, Switch/3
  注入时间/1 -> 使能/1
  使能/1 -> Switch/2

== system satellite3/姿态确定与控制系统/三轴姿态动力学子系统/陀螺仪故障/漂移故障 ==
  使能*幅度 : Gain  Gain=gyro_bias_on*gyro_drift_value
  注入时间 : simulink/Sources/Ramp  slope=1  start=gyro_drift_time  InitialOutput=0
  限幅 : Saturate  UpperLimit=gyro_drift_max  LowerLimit=-gyro_drift_max
  故障值注入 : Outport
  wires:
  使能*幅度/1 -> 限幅/1
  注入时间/1 -> 使能*幅度/1
  限幅/1 -> 故障值注入/1

== system satellite3/姿态确定与控制系统/三轴姿态动力学子系统/陀螺仪故障/锁死故障 ==
  原值 : Inport
  Switch : Switch  Criteria=u2 > Threshold  Threshold=0.5  SaturateOnIntegerOverflow=off  InputSameDT=off
  上一值 : UnitDelay  SampleTime=-1  HasFrameUpgradeWarning=on
  使能 : Gain  Gain=gyro_lock_on
  抵消 : Sum  Inputs=|+-
  注入时间 : Step  Time=gyro_lock_time  SampleTime=0
  故障值注入 : Outport
  wires:
  注入时间/1 -> 使能/1
  抵消/1 -> 故障值注入/1
  上一值/1 -> Switch/1
  使能/1 -> Switch/2
  原值/1 -> Switch/3, 抵消/2
  Switch/1 -> 上一值/1, 抵消/1

== system satellite3/姿态确定与控制系统/金字塔反作用轮组件/反作用轮组件/反作用轮1 ==
  指令力矩 : Inport
  Bus Creator : BusCreator  Inputs=4  OutDataTypeStr=Bus: wheel1
  Integrator Limited : Integrator  LimitOutput=on  UpperSaturationLimit=1  LowerSaturationLimit=0
  Ki_tau : Gain  Gain=ki_w
  Kp_tau : Gain  Gain=kp_w
  Scope : Scope
      settings: ActiveDisplayYMinimum=-0.012901771580922018  ActiveDisplayYMaximum=0.009125331023455821  DataLoggingVariableName=ScopeData30
  Scope1 : Scope
      settings: DataLoggingVariableName=ScopeData37
  Sum : Sum  Inputs=|+-
  Sum1 : Sum  Inputs=|++
  Sum2 : Sum  Inputs=|+-
  力矩限幅 : Saturate  UpperLimit=T_max  LowerLimit=-T_max
  摩擦模型 : Subsystem
  期望电流限幅 : Saturate  UpperLimit=i_w_max  LowerLimit=i_w_min
  电流环等效 : TransferFcn  Denominator=[0.01 1]
  电磁转矩系数 : Gain  Gain=Cm
  轮力矩故障 : Subsystem
  轮摩擦故障 : Subsystem
  轮状态解算 : Subsystem
  Wheel : Outport
  wires:
  Sum/1 -> Kp_tau/1, Ki_tau/1
  电磁转矩系数/1 -> 轮力矩故障/1(原值)
  Kp_tau/1 -> Sum1/1
  指令力矩/1 -> Sum/1
  Integrator Limited/1 -> Sum1/2
  Ki_tau/1 -> Integrator Limited/1
  Sum1/1 -> 期望电流限幅/1
  期望电流限幅/1 -> 电流环等效/1
  Sum2/1 -> Bus Creator/2, Sum/2, 轮状态解算/1(作用力矩)  "tau"
  电流环等效/1 -> Bus Creator/1, 电磁转矩系数/1  "i"
  轮状态解算/1(转速) -> Bus Creator/3, Scope/1, 摩擦模型/1(转速)  "n"
  Bus Creator/1 -> Wheel/1
  轮状态解算/2(角动量) -> Bus Creator/4  "h"
  摩擦模型/1(摩擦力矩) -> 轮摩擦故障/1(原值)
  轮力矩故障/1(故障值) -> 力矩限幅/1
  力矩限幅/1 -> Sum2/1  "tau"
  轮摩擦故障/1(故障值) -> Scope1/1, Sum2/2

== system satellite3/姿态确定与控制系统/金字塔反作用轮组件/反作用轮组件/反作用轮2 ==
  指令力矩 : Inport
  Bus Creator : BusCreator  Inputs=4  OutDataTypeStr=Bus: wheel1
  Integrator Limited : Integrator  LimitOutput=on  UpperSaturationLimit=1  LowerSaturationLimit=0
  Ki_tau : Gain  Gain=ki_w
  Kp_tau : Gain  Gain=kp_w
  Scope : Scope
      settings: ActiveDisplayYMinimum=-0.012901771580922018  ActiveDisplayYMaximum=0.009125331023455821  DataLoggingVariableName=ScopeData30
  Scope1 : Scope
      settings: DataLoggingVariableName=ScopeData37
  Sum : Sum  Inputs=|+-
  Sum1 : Sum  Inputs=|++
  Sum2 : Sum  Inputs=|+-
  力矩限幅 : Saturate  UpperLimit=T_max  LowerLimit=-T_max
  摩擦模型 : Subsystem
  期望电流限幅 : Saturate  UpperLimit=i_w_max  LowerLimit=i_w_min
  电流环等效 : TransferFcn  Denominator=[0.01 1]
  电磁转矩系数 : Gain  Gain=Cm
  轮力矩故障 : Subsystem
  轮摩擦故障 : Subsystem
  轮状态解算 : Subsystem
  Wheel : Outport
  wires:
  力矩限幅/1 -> Sum2/1  "tau"
  轮力矩故障/1(故障值) -> 力矩限幅/1
  摩擦模型/1(摩擦力矩) -> 轮摩擦故障/1(原值)
  轮状态解算/2(角动量) -> Bus Creator/4  "h"
  Bus Creator/1 -> Wheel/1
  轮状态解算/1(转速) -> 摩擦模型/1(转速), Scope/1, Bus Creator/3  "n"
  电流环等效/1 -> 电磁转矩系数/1, Bus Creator/1  "i"
  Sum2/1 -> 轮状态解算/1(作用力矩), Sum/2, Bus Creator/2  "tau"
  期望电流限幅/1 -> 电流环等效/1
  Sum1/1 -> 期望电流限幅/1
  Ki_tau/1 -> Integrator Limited/1
  Integrator Limited/1 -> Sum1/2
  指令力矩/1 -> Sum/1
  Kp_tau/1 -> Sum1/1
  电磁转矩系数/1 -> 轮力矩故障/1(原值)
  Sum/1 -> Ki_tau/1, Kp_tau/1
  轮摩擦故障/1(故障值) -> Sum2/2, Scope1/1

== system satellite3/姿态确定与控制系统/金字塔反作用轮组件/反作用轮组件/反作用轮3 ==
  指令力矩 : Inport
  Bus Creator : BusCreator  Inputs=4  OutDataTypeStr=Bus: wheel1
  Integrator Limited : Integrator  LimitOutput=on  UpperSaturationLimit=1  LowerSaturationLimit=0
  Ki_tau : Gain  Gain=ki_w
  Kp_tau : Gain  Gain=kp_w
  Scope : Scope
      settings: ActiveDisplayYMinimum=-0.012901771580922018  ActiveDisplayYMaximum=0.009125331023455821  DataLoggingVariableName=ScopeData30
  Scope1 : Scope
      settings: DataLoggingVariableName=ScopeData37
  Sum : Sum  Inputs=|+-
  Sum1 : Sum  Inputs=|++
  Sum2 : Sum  Inputs=|+-
  力矩限幅 : Saturate  UpperLimit=T_max  LowerLimit=-T_max
  摩擦模型 : Subsystem
  期望电流限幅 : Saturate  UpperLimit=i_w_max  LowerLimit=i_w_min
  电流环等效 : TransferFcn  Denominator=[0.01 1]
  电磁转矩系数 : Gain  Gain=Cm
  轮力矩故障 : Subsystem
  轮摩擦故障 : Subsystem
  轮状态解算 : Subsystem
  Wheel : Outport
  wires:
  Sum/1 -> Kp_tau/1, Ki_tau/1
  电磁转矩系数/1 -> 轮力矩故障/1(原值)
  Kp_tau/1 -> Sum1/1
  指令力矩/1 -> Sum/1
  Integrator Limited/1 -> Sum1/2
  Ki_tau/1 -> Integrator Limited/1
  Sum1/1 -> 期望电流限幅/1
  期望电流限幅/1 -> 电流环等效/1
  Sum2/1 -> Bus Creator/2, Sum/2, 轮状态解算/1(作用力矩)  "tau"
  电流环等效/1 -> Bus Creator/1, 电磁转矩系数/1  "i"
  轮状态解算/1(转速) -> Bus Creator/3, Scope/1, 摩擦模型/1(转速)  "n"
  Bus Creator/1 -> Wheel/1
  轮状态解算/2(角动量) -> Bus Creator/4  "h"
  摩擦模型/1(摩擦力矩) -> 轮摩擦故障/1(原值)
  轮力矩故障/1(故障值) -> 力矩限幅/1
  力矩限幅/1 -> Sum2/1  "tau"
  轮摩擦故障/1(故障值) -> Sum2/2, Scope1/1

== system satellite3/姿态确定与控制系统/金字塔反作用轮组件/反作用轮组件/反作用轮4 ==
  指令力矩 : Inport
  Bus Creator : BusCreator  Inputs=4  OutDataTypeStr=Bus: wheel1
  Integrator Limited : Integrator  LimitOutput=on  UpperSaturationLimit=1  LowerSaturationLimit=0
  Ki_tau : Gain  Gain=ki_w
  Kp_tau : Gain  Gain=kp_w
  Scope : Scope
      settings: ActiveDisplayYMinimum=-0.012901771580922018  ActiveDisplayYMaximum=0.009125331023455821  DataLoggingVariableName=ScopeData30
  Scope1 : Scope
      settings: DataLoggingVariableName=ScopeData37
  Sum : Sum  Inputs=|+-
  Sum1 : Sum  Inputs=|++
  Sum2 : Sum  Inputs=|+-
  力矩限幅 : Saturate  UpperLimit=T_max  LowerLimit=-T_max
  摩擦模型 : Subsystem
  期望电流限幅 : Saturate  UpperLimit=i_w_max  LowerLimit=i_w_min
  电流环等效 : TransferFcn  Denominator=[0.01 1]
  电磁转矩系数 : Gain  Gain=Cm
  轮力矩故障 : Subsystem
  轮摩擦故障 : Subsystem
  轮状态解算 : Subsystem
  Wheel : Outport
  wires:
  力矩限幅/1 -> Sum2/1  "tau"
  轮力矩故障/1(故障值) -> 力矩限幅/1
  摩擦模型/1(摩擦力矩) -> 轮摩擦故障/1(原值)
  轮状态解算/2(角动量) -> Bus Creator/4  "h"
  Bus Creator/1 -> Wheel/1
  轮状态解算/1(转速) -> 摩擦模型/1(转速), Scope/1, Bus Creator/3  "n"
  电流环等效/1 -> 电磁转矩系数/1, Bus Creator/1  "i"
  Sum2/1 -> 轮状态解算/1(作用力矩), Sum/2, Bus Creator/2  "tau"
  期望电流限幅/1 -> 电流环等效/1
  Sum1/1 -> 期望电流限幅/1
  Ki_tau/1 -> Integrator Limited/1
  Integrator Limited/1 -> Sum1/2
  指令力矩/1 -> Sum/1
  Kp_tau/1 -> Sum1/1
  电磁转矩系数/1 -> 轮力矩故障/1(原值)
  Sum/1 -> Ki_tau/1, Kp_tau/1
  轮摩擦故障/1(故障值) -> Scope1/1, Sum2/2

== system satellite3/推进子系统/化推/推力故障/延迟故障 ==
  原值 : Inport
  Delay : Delay  DelayLength=cT_delay_value
  Switch : Switch  Criteria=u2 > Threshold  Threshold=0.5  SaturateOnIntegerOverflow=off  InputSameDT=off
  使能 : Gain  Gain=cT_delay_on
  抵消 : Sum  Inputs=|+-
  注入时间 : Step  Time=cT_delay_time  SampleTime=0
  故障值注入 : Outport
  wires:
  Delay/1 -> Switch/1
  Switch/1 -> 抵消/1
  抵消/1 -> 故障值注入/1
  原值/1 -> 抵消/2, Delay/1, Switch/3
  注入时间/1 -> 使能/1
  使能/1 -> Switch/2

== system satellite3/推进子系统/化推/推力故障/掉线故障 ==
  原值 : Inport
  Switch : Switch  Criteria=u2 > Threshold  Threshold=0.5  SaturateOnIntegerOverflow=off  InputSameDT=off
  Zero : Constant  Value=cT_drop_value  OutDataTypeStr=Inherit: Inherit via back propagation
  使能 : Gain  Gain=cT_drop_on
  抵消 : Sum  Inputs=|+-
  注入时间 : Step  Time=cT_drop_time  SampleTime=0
  故障值注入 : Outport
  wires:
  使能/1 -> Switch/2
  注入时间/1 -> 使能/1
  原值/1 -> Switch/3, 抵消/2
  抵消/1 -> 故障值注入/1
  Switch/1 -> 抵消/1
  Zero/1 -> Switch/1

== system satellite3/推进子系统/化推/推力故障/退化故障 ==
  原值 : Inport
  Switch : Switch  Criteria=u2 > Threshold  Threshold=0.5  SaturateOnIntegerOverflow=off  InputSameDT=off
  使能 : Gain  Gain=cT_deg_on
  幅度 : Gain  Gain=cT_deg_value
  抵消 : Sum  Inputs=|+-
  注入时间 : Step  Time=cT_deg_time  SampleTime=0
  故障值注入 : Outport
  wires:
  Switch/1 -> 抵消/1
  原值/1 -> 抵消/2, 幅度/1, Switch/3
  使能/1 -> Switch/2
  抵消/1 -> 故障值注入/1
  注入时间/1 -> 使能/1
  幅度/1 -> Switch/1

== system satellite3/推进子系统/化推/推力故障/锁死故障 ==
  原值 : Inport
  Switch : Switch  Criteria=u2 > Threshold  Threshold=0.5  SaturateOnIntegerOverflow=off  InputSameDT=off
  上一值 : UnitDelay  SampleTime=-1  HasFrameUpgradeWarning=on
  使能 : Gain  Gain=cT_lock_on
  抵消 : Sum  Inputs=|+-
  注入时间 : Step  Time=cT_lock_time  SampleTime=0
  故障值注入 : Outport
  wires:
  Switch/1 -> 抵消/1, 上一值/1
  原值/1 -> 抵消/2, Switch/3
  使能/1 -> Switch/2
  上一值/1 -> Switch/1
  抵消/1 -> 故障值注入/1
  注入时间/1 -> 使能/1

== system satellite3/推进子系统/电推/推力故障/延迟故障 ==
  原值 : Inport
  Delay : Delay  DelayLength=eT_delay_value
  Switch : Switch  Criteria=u2 > Threshold  Threshold=0.5  SaturateOnIntegerOverflow=off  InputSameDT=off
  使能 : Gain  Gain=eT_delay_on
  抵消 : Sum  Inputs=|+-
  注入时间 : Step  Time=eT_delay_time  SampleTime=0
  故障值注入 : Outport
  wires:
  Delay/1 -> Switch/1
  Switch/1 -> 抵消/1
  抵消/1 -> 故障值注入/1
  原值/1 -> 抵消/2, Delay/1, Switch/3
  注入时间/1 -> 使能/1
  使能/1 -> Switch/2

== system satellite3/推进子系统/电推/推力故障/掉线故障 ==
  原值 : Inport
  Switch : Switch  Criteria=u2 > Threshold  Threshold=0.5  SaturateOnIntegerOverflow=off  InputSameDT=off
  Zero : Constant  Value=eT_drop_value  OutDataTypeStr=Inherit: Inherit via back propagation
  使能 : Gain  Gain=eT_drop_on
  抵消 : Sum  Inputs=|+-
  注入时间 : Step  Time=eT_drop_time  SampleTime=0
  故障值注入 : Outport
  wires:
  使能/1 -> Switch/2
  注入时间/1 -> 使能/1
  原值/1 -> Switch/3, 抵消/2
  抵消/1 -> 故障值注入/1
  Switch/1 -> 抵消/1
  Zero/1 -> Switch/1

== system satellite3/推进子系统/电推/推力故障/退化故障 ==
  原值 : Inport
  Switch : Switch  Criteria=u2 > Threshold  Threshold=0.5  SaturateOnIntegerOverflow=off  InputSameDT=off
  使能 : Gain  Gain=eT_deg_on
  幅度 : Gain  Gain=eT_deg_value
  抵消 : Sum  Inputs=|+-
  注入时间 : Step  Time=eT_deg_time  SampleTime=0
  故障值注入 : Outport
  wires:
  Switch/1 -> 抵消/1
  原值/1 -> 抵消/2, 幅度/1, Switch/3
  使能/1 -> Switch/2
  抵消/1 -> 故障值注入/1
  注入时间/1 -> 使能/1
  幅度/1 -> Switch/1

== system satellite3/推进子系统/电推/推力故障/锁死故障 ==
  原值 : Inport
  Switch : Switch  Criteria=u2 > Threshold  Threshold=0.5  SaturateOnIntegerOverflow=off  InputSameDT=off
  上一值 : UnitDelay  SampleTime=-1  HasFrameUpgradeWarning=on
  使能 : Gain  Gain=eT_lock_on
  抵消 : Sum  Inputs=|+-
  注入时间 : Step  Time=eT_lock_time  SampleTime=0
  故障值注入 : Outport
  wires:
  Switch/1 -> 抵消/1, 上一值/1
  原值/1 -> 抵消/2, Switch/3
  使能/1 -> Switch/2
  上一值/1 -> Switch/1
  抵消/1 -> 故障值注入/1
  注入时间/1 -> 使能/1

== system satellite3/测控子系统/视线角标志/余弦夹角/向量模长-r1 ==
  u1 : Inport
  u2 : Inport  Port=2
  u3 : Inport  Port=3
  Add : Sum  Inputs=+++
  Sqrt : Sqrt
  Square : Math  Operator=square
  Square1 : Math  Operator=square
  Square2 : Math  Operator=square
  |u| : Outport
  wires:
  Sqrt/1 -> |u|/1
  Add/1 -> Sqrt/1
  Square2/1 -> Add/3
  Square1/1 -> Add/2
  Square/1 -> Add/1
  u3/1 -> Square2/1
  u2/1 -> Square1/1
  u1/1 -> Square/1

== system satellite3/测控子系统/视线角标志/余弦夹角/向量模长-r2 ==
  u1 : Inport
  u2 : Inport  Port=2
  u3 : Inport  Port=3
  Add : Sum  Inputs=+++
  Sqrt : Sqrt
  Square : Math  Operator=square
  Square1 : Math  Operator=square
  Square2 : Math  Operator=square
  |u| : Outport
  wires:
  u1/1 -> Square/1
  u2/1 -> Square1/1
  u3/1 -> Square2/1
  Square/1 -> Add/1
  Square1/1 -> Add/2
  Square2/1 -> Add/3
  Add/1 -> Sqrt/1
  Sqrt/1 -> |u|/1

== system satellite3/电源子系统/太阳能板/太阳板/伏电特性 ==
  note: $I=(N_p\cdot I_{ph})-(N_p\cdot I_0)\left(e^{\frac{V+I(N_s\cdot R_s / N_p)}{(N_s\cdot n)V_t}}-1\right)-\frac{V+I(N_s\cdot R_s / N_p)}{N_s\cdot R_{sh} / N_p}$
  lr : Inport
  V : Inport  Port=2
  Controlled Voltage Source : fl_lib/Electrical/Electrical Sources/Controlled Voltage Source
  ERef : fl_lib/Electrical/Electrical Elements/Electrical Reference
  Sensing Current : Subsystem
      mask Display: disp('i')
  Simulink-PS Converter : nesl_utility/Simulink-PS Converter  PhysicalDomain=network_engine_domain  SubClassName=ps_input  LeftPortType=input  RightPortType=output  PseudoPeriodic=off  Frequencies=[]  NoiseDistribution=none  NoiseParameters=[]  Unit=W/m^2  AffineConversion=off  FilteringAndDerivatives=provide  SimscapeFilterOrder=1  InputFilterTimeConstant=0.01  UdotUserProvided=0
  Simulink-PS Converter1 : nesl_utility/Simulink-PS Converter  PhysicalDomain=network_engine_domain  SubClassName=ps_input  LeftPortType=input  RightPortType=output  PseudoPeriodic=off  Frequencies=[]  NoiseDistribution=none  NoiseParameters=[]  Unit=1  AffineConversion=off  FilteringAndDerivatives=zero  SimscapeFilterOrder=1  InputFilterTimeConstant=0.001  UdotUserProvided=1
  Solar Cell1 : ee_lib/Sources/Solar Cell  prm=ee.enum.sources.solar_cell_prm.eightParameter  Isc=3.8 A  Voc=0.586 V  Is=I_f A  Is2=0 A  Iph=I_sc A  Ir0=G0 W/m^2  ec=n_diode  N2=2  Rs=R_s Ohm  Rp=R_p Ohm  N_series=num_s  N_parallel=num_p  TIPH1=0.000805 1/K  EG=1.14 eV  TXIS1=3.38  TXIS2=3  TRS1=0  TRP1=0  Tmeas=25 degC  TFIXED=25 degC  thermal_mass=100 J/K  initial_temperature=25 degC
  Solver Configuration : nesl_utility/Solver Configuration  PhysicalDomain=network_engine_domain  SubClassName=solver  LeftPortType=input  RightPortType=generic  Tones=[]  Harmonics=[]  SimulateNoise=off  Profile=off  UseLocalSampling=off  EnableSwitchedLinearOptims=on  FrequencyDomain=off  UseCCode=off  RelTol=0.001  AbsTol=1e-06  MinStep=1e-09  ToWorkspace=off  RevertToSquareIcSolve=off  NumHomotopyIterations=100  PhasorMode=off  PhasorModeNumHarmonics=1  ConsistencySolver=NEWTON_FTOL  IndexReductionMethod=DerivativeReplacement  DoDC=off  ResidualTolerance=1e-9  ConsistencyTolSource=GLOBAL  ConsistencyAbsTol=0.001  ConsistencyRelTol=0.001  ConsistencyTolFactor=0.001  UseLocalSolver=off  LocalSolverChoice=NE_BACKWARD_EULER_ADVANCER  ResolveIndetEquations=on  FunctionEvalNumThread=1  LocalSolverSampleTime=0.1  DoFixedCost=off  MaxNonlinIter=3  MaxModeIter=2  ComputeImpulses=off  ImpulseIterations=2  LinearAlgebra=auto  LinearAlgebraNumThread=0  EquationFormulation=NE_TIME_EF  DelaysMemoryBudget=1024  AutomaticFiltering=on  FilteringTimeConstant=0.001  PartitionStorageMethod=AS_NEEDED  PartitionMemoryBudget=1024  PartitionMethod=FAST  MultibodyUseLocalSolver=off  MultibodyLocalSolverChoice=ODE1  MultibodyLocalSolverSampleTime=0.001
  I : Outport
  wires:
  lr/1 -> Simulink-PS Converter/1
  Sensing Current/1(Out1) -> I/1
  V/1 -> Simulink-PS Converter1/1
  connections:
  Simulink-PS Converter/RConn1 -- Solar Cell1/LConn1
  Sensing Current/LConn1 -- Solar Cell1/LConn2
  Simulink-PS Converter1/RConn1 -- Controlled Voltage Source/RConn1
  Controlled Voltage Source/LConn1 -- Sensing Current/RConn1
  Controlled Voltage Source/RConn2 -- ERef/LConn1 -- Solar Cell1/RConn1 -- Solver Configuration/RConn1

== system satellite3/电源子系统/太阳能板/太阳板/入射角余弦 ==
  note: $\hat{s}_b=q^*\otimes\hat{s}_i\otimes q$ 取矢量部分
  q : Inport
  星日单位矢量 : Inport  Port=2
  Max : MinMax  Function=max  Inputs=2
  Scope : Scope
      settings: ActiveDisplayYMinimum=-2.2349528929678062  ActiveDisplayYMaximum=1.7828322750992502  DataLoggingVariableName=ScopeData19
  Scope1 : Scope
      settings: ActiveDisplayYMinimum=-0.1208332283667245  ActiveDisplayYMaximum=1.0874990553005208  DataLoggingVariableName=ScopeData45
  Scope3 : Scope
      settings: ActiveDisplayYMinimum=-1.2077864910553922  ActiveDisplayYMaximum=1.1477558437901816  DataLoggingVariableName=ScopeData44
  Vector Concatenate : Concatenate  Mode=Multidimensional array
  余弦夹角 : Subsystem
  共轭 : Subsystem
  四元数乘法 : Subsystem
  四元数旋转 : Subsystem
  面板法向量 : Constant  Value=n_solar
  入射角余弦 : Outport
  wires:
  四元数旋转/1(Q*) -> Scope/1, 余弦夹角/2(u2)
  四元数乘法/1(Q*) -> 四元数旋转/1(Q1)
  q/1 -> 四元数旋转/2(Q2), 共轭/1(q)
  面板法向量/1 -> 余弦夹角/1(u1)
  共轭/1(q*) -> 四元数乘法/1(Q1)
  Max/1 -> Scope1/1, 入射角余弦/1
  [zero] -> Vector Concatenate/1, Max/2
  Vector Concatenate/1 -> 四元数乘法/2(Q2)
  余弦夹角/1(cos(γ)) -> Scope3/1, Max/1
  星日单位矢量/1 -> Vector Concatenate/2

== system satellite3/电源子系统/太阳能板/太阳板/太阳翼故障 ==
  原值 : Inport
  Add : Sum  Inputs=2
  Sum : Sum  Inputs=|++
  掉线故障 : Subsystem
  退化故障 : Subsystem
  故障值 : Outport
  wires:
  退化故障/1(故障值注入) -> Add/1
  Add/1 -> Sum/2
  Sum/1 -> 故障值/1
  原值/1 -> Sum/1, 掉线故障/1(原值), 退化故障/1(原值)
  掉线故障/1(故障值注入) -> Add/2

== system satellite3/电源子系统/太阳能板/太阳板/步进MPPT ==
  note: dP和dV同符号
  note: $I=(N_p\cdot I_{ph})-(N_p\cdot I_0)\left(e^{\frac{V+I(N_s\cdot R_s / N_p)}{(N_s\cdot n)V_t}}-1\right)-\frac{V+I(N_s\cdot R_s / N_p)}{N_s\cdot R_{sh} / N_p}$
  I_panel : Inport
  母线电压 : Inport  Port=2
  Abs : Abs  SaturateOnIntegerOverflow=off
  Add1 : Sum
  Constant : Constant  Value=D_max
  D_sat : simulink/Discontinuities/Saturation Dynamic  OutMin=[]  OutMax=[D_max]  OutDataTypeStr=Inherit: Same as second input  OutDataType=fixdt(1, 16)  OutScaling=2^-10  DoSatur=off
  Delta_D : Constant  Value=Delta_D*10
  Gain : Gain  Gain=-1
  Gain1 : Gain
  Product : Product
  Product1 : Product
  Product3 : Product
  Product5 : Product  Inputs=*/
  Saturation : Saturate  UpperLimit=1  LowerLimit=0
  Scope : Scope
      settings: ActiveDisplayYMinimum=-27.136387311423995  ActiveDisplayYMaximum=59.659571746199781  DataLoggingVariableName=ScopeData7
  Scope1 : Scope  NumInputPorts=2
      settings: ActiveDisplayYMinimum=0.56859420431681085  ActiveDisplayYMaximum=1.1751476631569284  DataLoggingVariableName=ScopeData50
  Sign : Signum
  Switch : Switch  SaturateOnIntegerOverflow=off  InputSameDT=off
  Switch1 : Switch  Criteria=u2 > Threshold  Threshold=dP_th  SaturateOnIntegerOverflow=off  InputSameDT=off
  UD_D : UnitDelay  InitialCondition=0.5  SampleTime=-1  HasFrameUpgradeWarning=on
  UD_P : UnitDelay  SampleTime=-1  HasFrameUpgradeWarning=on
  UD_V : UnitDelay  SampleTime=-1  HasFrameUpgradeWarning=on
  dP : Sum  Inputs=|+-
  dV : Sum  Inputs=|+-
  面板开路电压 : Constant  Value=V_oc
  太阳电池电压 : Outport
  wires:
  Product5/1 -> Saturation/1
  UD_D/1 -> Product1/2, Add1/1, Scope1/2
  Switch/1 -> Switch1/1
  Product3/1 -> dP/1, UD_P/1
  Add1/1 -> D_sat/2  "D"
  dV/1 -> Product/1
  UD_V/1 -> dV/2
  UD_P/1 -> dP/2
  Gain1/1 -> Switch/1
  Abs/1 -> Switch1/2
  Saturation/1 -> D_sat/3
  Constant/1 -> D_sat/1
  dP/1 -> Abs/1, Product/2
  Delta_D/1 -> Gain1/1, Gain/1
  Product/1 -> Sign/1
  母线电压/1 -> Product1/1, Product5/1
  D_sat/1 -> UD_D/1, Scope1/1
  面板开路电压/1 -> Product5/2
  Gain/1 -> Switch/3
  [zero] -> Switch1/3
  Switch1/1 -> Add1/2
  Sign/1 -> Switch/2
  I_panel/1 -> Product3/1
  Product1/1 -> 太阳电池电压/1, Scope/1, Product3/2, UD_V/1, dV/1

== system satellite3/电源子系统/太阳能板/母线故障/偏差故障 ==
  使能*幅度 : Gain  Gain=Vbus_bias_on*Vbus_bias_value
  注入时间 : Step  Time=Vbus_bias_time  SampleTime=0
  故障值注入 : Outport
  wires:
  使能*幅度/1 -> 故障值注入/1
  注入时间/1 -> 使能*幅度/1

== system satellite3/电源子系统/太阳能板/母线故障/掉线故障 ==
  原值 : Inport
  Switch : Switch  Criteria=u2 > Threshold  Threshold=0.5  SaturateOnIntegerOverflow=off  InputSameDT=off
  Zero : Constant  Value=Vbus_drop_value  OutDataTypeStr=Inherit: Inherit via back propagation
  使能 : Gain  Gain=Vbus_drop_on
  抵消 : Sum  Inputs=|+-
  注入时间 : Step  Time=Vbus_drop_time  SampleTime=0
  故障值注入 : Outport
  wires:
  使能/1 -> Switch/2
  注入时间/1 -> 使能/1
  原值/1 -> Switch/3, 抵消/2
  抵消/1 -> 故障值注入/1
  Switch/1 -> 抵消/1
  Zero/1 -> Switch/1

== system satellite3/电源子系统/蓄电池组/蓄电池组故障/乘性故障 ==
  原值 : Inport
  Switch : Switch  Criteria=u2 > Threshold  Threshold=0.5  SaturateOnIntegerOverflow=off  InputSameDT=off
  使能 : Gain  Gain=bat_cap_on
  幅度 : Gain  Gain=bat_cap_value
  抵消 : Sum  Inputs=|+-
  注入时间 : Step  Time=bat_cap_time  SampleTime=0
  故障值注入 : Outport
  wires:
  Switch/1 -> 抵消/1
  原值/1 -> 抵消/2, 幅度/1, Switch/3
  使能/1 -> Switch/2
  抵消/1 -> 故障值注入/1
  注入时间/1 -> 使能/1
  幅度/1 -> Switch/1

== system satellite3/电源子系统/蓄电池组/蓄电池组故障/偏差故障 ==
  使能*幅度 : Gain  Gain=bat_bias_on*bat_bias_value
  注入时间 : Step  Time=bat_bias_time  SampleTime=0
  故障值注入 : Outport
  wires:
  使能*幅度/1 -> 故障值注入/1
  注入时间/1 -> 使能*幅度/1

== system satellite3/姿态确定与控制系统/三轴姿态动力学子系统/姿态解算/四元数传播-欧拉法/向量模长-q ==
  u0 : Inport
  u1 : Inport  Port=2
  u2 : Inport  Port=3
  u3 : Inport  Port=4
  Add : Sum  Inputs=4
  Sqrt : Sqrt
  Square{,1..3} (4 alike) : Math  Operator=square
  |u| : Outport
  wires:
  u0/1 -> Square/1
  u1/1 -> Square1/1
  u2/1 -> Square2/1
  Square/1 -> Add/1
  Square1/1 -> Add/2
  Square2/1 -> Add/3
  Add/1 -> Sqrt/1
  Sqrt/1 -> |u|/1
  u3/1 -> Square3/1
  Square3/1 -> Add/4

== system satellite3/姿态确定与控制系统/三轴姿态动力学子系统/姿态解算/星敏/四元数乘法 ==
  Q1 : Inport
  Q2 : Inport  Port=2
  Add : Sum  Inputs=3
  Cross Product : matrix_library/Cross Product
  Demux : Demux
  Demux1 : Demux
  Dot Product : DotProduct  OutDataTypeStr=Inherit: Inherit via internal rule
  Mux : Mux  Inputs=2
  Mux1 : Mux  Inputs=3
  Mux2 : Mux  Inputs=3
  Product : Product
  Product1 : Product
  Product2 : Product
  Sum : Sum  Inputs=|+-
  Q* : Outport
  wires:
  Q1/1 -> Demux/1
  Q2/1 -> Demux1/1
  Mux/1 -> Q*/1
  Product/1 -> Sum/1
  Demux/1 -> Product1/1, Product/1
  Mux1/1 -> Dot Product/1, Cross Product/1, Product2/2
  Demux1/1 -> Product2/1, Product/2
  Mux2/1 -> Cross Product/2, Dot Product/2, Product1/2
  Sum/1 -> Mux/1
  Dot Product/1 -> Sum/2
  Product2/1 -> Add/2
  Product1/1 -> Add/1
  Cross Product/1 -> Add/3
  Add/1 -> Mux/2
  Demux/2 -> Mux1/1
  Demux/3 -> Mux1/2
  Demux/4 -> Mux1/3
  Demux1/2 -> Mux2/1
  Demux1/3 -> Mux2/2
  Demux1/4 -> Mux2/3

== system satellite3/姿态确定与控制系统/三轴姿态动力学子系统/姿态解算/星敏/四元数归一化 ==
  Q* : Inport
  Demux1 : Demux
  Mux1 : Mux
  Product{2..5} (4 alike) : Product  Inputs=*/
  向量模长-q : Subsystem
  Out1 : Outport
  wires:
  Demux1/4 -> Product5/1, 向量模长-q/4(u3)
  Product5/1 -> Mux1/4  "q3"
  Demux1/2 -> 向量模长-q/2(u1), Product3/1
  向量模长-q/1(|u|) -> Product3/2, Product4/2, Product5/2, Product2/2
  Demux1/1 -> 向量模长-q/1(u0), Product2/1
  Demux1/3 -> 向量模长-q/3(u2), Product4/1
  Product3/1 -> Mux1/2  "q1"
  Product2/1 -> Mux1/1  "q0"
  Product4/1 -> Mux1/3  "q2"
  Mux1/1 -> Out1/1
  Q*/1 -> Demux1/1

== system satellite3/姿态确定与控制系统/三轴姿态动力学子系统/姿态解算/星敏/误差四元数 ==
  note: 先用正弦伪噪声，再考虑换成随机噪声
  1 : simulink/Sources/Band-Limited White Noise  Cov=[0.1]  Ts=0.1  seed=[23341]
  Mux : Mux
  Sine Wave : Sin  Amplitude=sigma_rad/2  Frequency=2*pi*1  SampleTime=0
  Sine Wave1 : Sin  Amplitude=sigma_rad/2  Frequency=2*pi*1  SampleTime=0
  Sine Wave2 : Sin  Amplitude=sigma_rad/2  Frequency=2*pi*1  SampleTime=0
  delta_q : Outport
  wires:
  Sine Wave2/1 -> Mux/4
  [one] -> Mux/1
  Sine Wave/1 -> Mux/2
  Mux/1 -> delta_q/1
  Sine Wave1/1 -> Mux/3

== system satellite3/姿态确定与控制系统/三轴姿态动力学子系统/姿态解算/简化互补滤波器/共轭 ==
  u : Inport
  -q1 : Gain  Gain=-1
  -q2 : Gain  Gain=-1
  -q3 : Gain  Gain=-1
  Demux : Demux
  Mux : Mux
  u^-1 : Outport
  wires:
  Mux/1 -> u^-1/1
  Demux/1 -> Mux/1
  Demux/2 -> -q1/1
  -q1/1 -> Mux/2
  Demux/3 -> -q2/1
  -q2/1 -> Mux/3
  Demux/4 -> -q3/1
  -q3/1 -> Mux/4
  u/1 -> Demux/1
